simulink model "showKeyPoint"  (R2015a)
settings: Solver=ode45  StartTime=0.0  StopTime=10.0  RelTol=1e-3
InitFcn:
  | %% DSPBuilder Start
  | alt_dspbuilder_update_model(bdroot)
  | %% DSPBuilder End
libraries: allblocks_alteradspbuilder2 x340
(part 2 of 5)

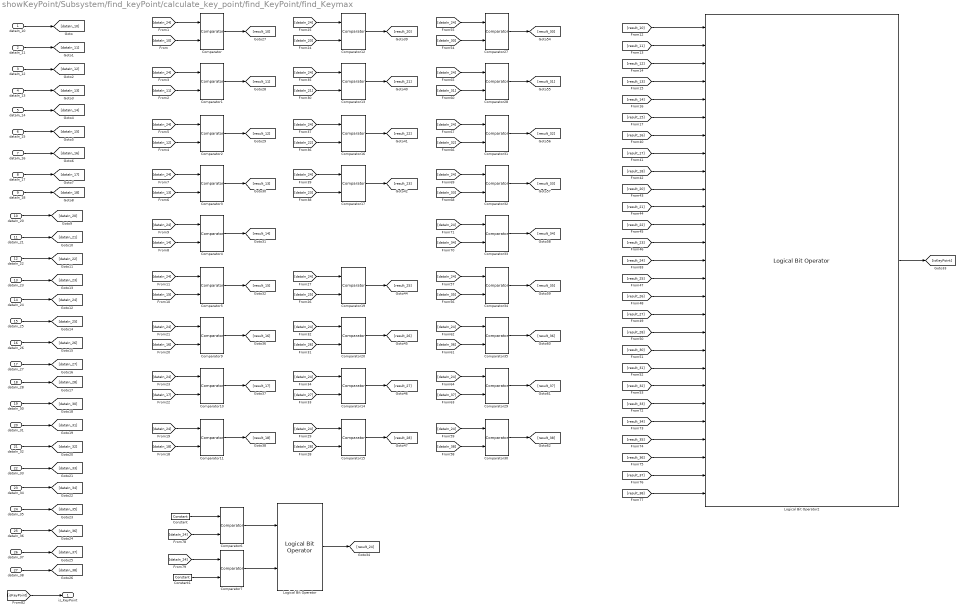
== system showKeyPoint/Subsystem/find_keyPoint/calculate_key_point/find_KeyPoint/find_Keymax ==
  dataIn_10 : Inport
  dataIn_11 : Inport  Port=2
  dataIn_12 : Inport  Port=3
  dataIn_13 : Inport  Port=4
  dataIn_14 : Inport  Port=5
  dataIn_15 : Inport  Port=6
  dataIn_16 : Inport  Port=7
  dataIn_17 : Inport  Port=8
  dataIn_18 : Inport  Port=9
  dataIn_20 : Inport  Port=10
  dataIn_21 : Inport  Port=11
  dataIn_22 : Inport  Port=12
  dataIn_23 : Inport  Port=13
  dataIn_24 : Inport  Port=14
  dataIn_25 : Inport  Port=15
  dataIn_26 : Inport  Port=16
  dataIn_27 : Inport  Port=17
  dataIn_28 : Inport  Port=18
  dataIn_30 : Inport  Port=19
  dataIn_31 : Inport  Port=20
  dataIn_32 : Inport  Port=21
  dataIn_33 : Inport  Port=22
  dataIn_34 : Inport  Port=23
  dataIn_35 : Inport  Port=24
  dataIn_36 : Inport  Port=25
  dataIn_37 : Inport  Port=26
  dataIn_38 : Inport  Port=27
  Comparator : allblocks_alteradspbuilder2/Comparator  direction=a > b  pipeline_display=0  allowFloatingPointOverride=on  logOutputs=off  logFile=C:\Users\ASUS\Desktop\sift_fpga_final\Gaussian filter 5x5\tb_gauss\gauss_Subsystem_find%5FkeyPoint_calculate%5Fkey%5Fpoint_find%5FKeyPoint_find%5FKeymax_Comparator.fixedpointlog
  Comparator1 : allblocks_alteradspbuilder2/Comparator  direction=a > b  pipeline_display=0  allowFloatingPointOverride=on  logOutputs=off  logFile=C:\Users\ASUS\Desktop\sift_fpga_final\Gaussian filter 5x5\tb_gauss\gauss_Subsystem_find%5FkeyPoint_calculate%5Fkey%5Fpoint_find%5FKeyPoint_find%5FKeymax_Comparator1.fixedpointlog
  Comparator10 : allblocks_alteradspbuilder2/Comparator  direction=a > b  pipeline_display=0  allowFloatingPointOverride=on  logOutputs=off  logFile=C:\Users\ASUS\Desktop\sift_fpga_final\Gaussian filter 5x5\tb_gauss\gauss_Subsystem_find%5FkeyPoint_calculate%5Fkey%5Fpoint_find%5FKeyPoint_find%5FKeymax_Comparator10.fixedpointlog
  Comparator11 : allblocks_alteradspbuilder2/Comparator  direction=a > b  pipeline_display=0  allowFloatingPointOverride=on  logOutputs=off  logFile=C:\Users\ASUS\Desktop\sift_fpga_final\Gaussian filter 5x5\tb_gauss\gauss_Subsystem_find%5FkeyPoint_calculate%5Fkey%5Fpoint_find%5FKeyPoint_find%5FKeymax_Comparator11.fixedpointlog
  Comparator12 : allblocks_alteradspbuilder2/Comparator  direction=a > b  pipeline_display=0  allowFloatingPointOverride=on  logOutputs=off  logFile=C:\Users\ASUS\Desktop\sift_fpga_final\Gaussian filter 5x5\tb_gauss\gauss_Subsystem_find%5FkeyPoint_calculate%5Fkey%5Fpoint_find%5FKeyPoint_find%5FKeymax_Comparator12.fixedpointlog
  Comparator13 : allblocks_alteradspbuilder2/Comparator  direction=a > b  pipeline_display=0  allowFloatingPointOverride=on  logOutputs=off  logFile=C:\Users\ASUS\Desktop\sift_fpga_final\Gaussian filter 5x5\tb_gauss\gauss_Subsystem_find%5FkeyPoint_calculate%5Fkey%5Fpoint_find%5FKeyPoint_find%5FKeymax_Comparator13.fixedpointlog
  Comparator14 : allblocks_alteradspbuilder2/Comparator  direction=a > b  pipeline_display=0  allowFloatingPointOverride=on  logOutputs=off  logFile=C:\Users\ASUS\Desktop\sift_fpga_final\Gaussian filter 5x5\tb_gauss\gauss_Subsystem_find%5FkeyPoint_calculate%5Fkey%5Fpoint_find%5FKeyPoint_find%5FKeymax_Comparator14.fixedpointlog
  Comparator15 : allblocks_alteradspbuilder2/Comparator  direction=a > b  pipeline_display=0  allowFloatingPointOverride=on  logOutputs=off  logFile=C:\Users\ASUS\Desktop\sift_fpga_final\Gaussian filter 5x5\tb_gauss\gauss_Subsystem_find%5FkeyPoint_calculate%5Fkey%5Fpoint_find%5FKeyPoint_find%5FKeymax_Comparator15.fixedpointlog
  Comparator16 : allblocks_alteradspbuilder2/Comparator  direction=a > b  pipeline_display=0  allowFloatingPointOverride=on  logOutputs=off  logFile=C:\Users\ASUS\Desktop\sift_fpga_final\Gaussian filter 5x5\tb_gauss\gauss_Subsystem_find%5FkeyPoint_calculate%5Fkey%5Fpoint_find%5FKeyPoint_find%5FKeymax_Comparator16.fixedpointlog
  Comparator17 : allblocks_alteradspbuilder2/Comparator  direction=a > b  pipeline_display=0  allowFloatingPointOverride=on  logOutputs=off  logFile=C:\Users\ASUS\Desktop\sift_fpga_final\Gaussian filter 5x5\tb_gauss\gauss_Subsystem_find%5FkeyPoint_calculate%5Fkey%5Fpoint_find%5FKeyPoint_find%5FKeymax_Comparator17.fixedpointlog
  Comparator19 : allblocks_alteradspbuilder2/Comparator  direction=a > b  pipeline_display=0  allowFloatingPointOverride=on  logOutputs=off  logFile=C:\Users\ASUS\Desktop\sift_fpga_final\Gaussian filter 5x5\tb_gauss\gauss_Subsystem_find%5FkeyPoint_calculate%5Fkey%5Fpoint_find%5FKeyPoint_find%5FKeymax_Comparator19.fixedpointlog
  Comparator2 : allblocks_alteradspbuilder2/Comparator  direction=a > b  pipeline_display=0  allowFloatingPointOverride=on  logOutputs=off  logFile=C:\Users\ASUS\Desktop\sift_fpga_final\Gaussian filter 5x5\tb_gauss\gauss_Subsystem_find%5FkeyPoint_calculate%5Fkey%5Fpoint_find%5FKeyPoint_find%5FKeymax_Comparator2.fixedpointlog
  Comparator20 : allblocks_alteradspbuilder2/Comparator  direction=a > b  pipeline_display=0  allowFloatingPointOverride=on  logOutputs=off  logFile=C:\Users\ASUS\Desktop\sift_fpga_final\Gaussian filter 5x5\tb_gauss\gauss_Subsystem_find%5FkeyPoint_calculate%5Fkey%5Fpoint_find%5FKeyPoint_find%5FKeymax_Comparator20.fixedpointlog
  Comparator27 : allblocks_alteradspbuilder2/Comparator  direction=a > b  pipeline_display=0  allowFloatingPointOverride=on  logOutputs=off  logFile=C:\Users\ASUS\Desktop\sift_fpga_final\Gaussian filter 5x5\tb_gauss\gauss_Subsystem_find%5FkeyPoint_calculate%5Fkey%5Fpoint_find%5FKeyPoint_find%5FKeymax_Comparator27.fixedpointlog
  Comparator28 : allblocks_alteradspbuilder2/Comparator  direction=a > b  pipeline_display=0  allowFloatingPointOverride=on  logOutputs=off  logFile=C:\Users\ASUS\Desktop\sift_fpga_final\Gaussian filter 5x5\tb_gauss\gauss_Subsystem_find%5FkeyPoint_calculate%5Fkey%5Fpoint_find%5FKeyPoint_find%5FKeymax_Comparator28.fixedpointlog
  Comparator29 : allblocks_alteradspbuilder2/Comparator  direction=a > b  pipeline_display=0  allowFloatingPointOverride=on  logOutputs=off  logFile=C:\Users\ASUS\Desktop\sift_fpga_final\Gaussian filter 5x5\tb_gauss\gauss_Subsystem_find%5FkeyPoint_calculate%5Fkey%5Fpoint_find%5FKeyPoint_find%5FKeymax_Comparator29.fixedpointlog
  Comparator3 : allblocks_alteradspbuilder2/Comparator  direction=a > b  pipeline_display=0  allowFloatingPointOverride=on  logOutputs=off  logFile=C:\Users\ASUS\Desktop\sift_fpga_final\Gaussian filter 5x5\tb_gauss\gauss_Subsystem_find%5FkeyPoint_calculate%5Fkey%5Fpoint_find%5FKeyPoint_find%5FKeymax_Comparator3.fixedpointlog
  Comparator30 : allblocks_alteradspbuilder2/Comparator  direction=a > b  pipeline_display=0  allowFloatingPointOverride=on  logOutputs=off  logFile=C:\Users\ASUS\Desktop\sift_fpga_final\Gaussian filter 5x5\tb_gauss\gauss_Subsystem_find%5FkeyPoint_calculate%5Fkey%5Fpoint_find%5FKeyPoint_find%5FKeymax_Comparator30.fixedpointlog
  Comparator31 : allblocks_alteradspbuilder2/Comparator  direction=a > b  pipeline_display=0  allowFloatingPointOverride=on  logOutputs=off  logFile=C:\Users\ASUS\Desktop\sift_fpga_final\Gaussian filter 5x5\tb_gauss\gauss_Subsystem_find%5FkeyPoint_calculate%5Fkey%5Fpoint_find%5FKeyPoint_find%5FKeymax_Comparator31.fixedpointlog
  Comparator32 : allblocks_alteradspbuilder2/Comparator  direction=a > b  pipeline_display=0  allowFloatingPointOverride=on  logOutputs=off  logFile=C:\Users\ASUS\Desktop\sift_fpga_final\Gaussian filter 5x5\tb_gauss\gauss_Subsystem_find%5FkeyPoint_calculate%5Fkey%5Fpoint_find%5FKeyPoint_find%5FKeymax_Comparator32.fixedpointlog
  Comparator33 : allblocks_alteradspbuilder2/Comparator  direction=a > b  pipeline_display=0  allowFloatingPointOverride=on  logOutputs=off  logFile=C:\Users\ASUS\Desktop\sift_fpga_final\Gaussian filter 5x5\tb_gauss\gauss_Subsystem_find%5FkeyPoint_calculate%5Fkey%5Fpoint_find%5FKeyPoint_find%5FKeymax_Comparator33.fixedpointlog
  Comparator34 : allblocks_alteradspbuilder2/Comparator  direction=a > b  pipeline_display=0  allowFloatingPointOverride=on  logOutputs=off  logFile=C:\Users\ASUS\Desktop\sift_fpga_final\Gaussian filter 5x5\tb_gauss\gauss_Subsystem_find%5FkeyPoint_calculate%5Fkey%5Fpoint_find%5FKeyPoint_find%5FKeymax_Comparator34.fixedpointlog
  Comparator35 : allblocks_alteradspbuilder2/Comparator  direction=a > b  pipeline_display=0  allowFloatingPointOverride=on  logOutputs=off  logFile=C:\Users\ASUS\Desktop\sift_fpga_final\Gaussian filter 5x5\tb_gauss\gauss_Subsystem_find%5FkeyPoint_calculate%5Fkey%5Fpoint_find%5FKeyPoint_find%5FKeymax_Comparator35.fixedpointlog
  Comparator4 : allblocks_alteradspbuilder2/Comparator  direction=a > b  pipeline_display=0  allowFloatingPointOverride=on  logOutputs=off  logFile=C:\Users\ASUS\Desktop\sift_fpga_final\Gaussian filter 5x5\tb_gauss\gauss_Subsystem_find%5FkeyPoint_calculate%5Fkey%5Fpoint_find%5FKeyPoint_find%5FKeymax_Comparator4.fixedpointlog
  Comparator5 : allblocks_alteradspbuilder2/Comparator  direction=a > b  pipeline_display=0  allowFloatingPointOverride=on  logOutputs=off  logFile=C:\Users\ASUS\Desktop\sift_fpga_final\Gaussian filter 5x5\tb_gauss\gauss_Subsystem_find%5FkeyPoint_calculate%5Fkey%5Fpoint_find%5FKeyPoint_find%5FKeymax_Comparator5.fixedpointlog
  Comparator6 : allblocks_alteradspbuilder2/Comparator  direction=a < b  pipeline_display=0  allowFloatingPointOverride=on  logOutputs=off  logFile=C:\Users\ASUS\Desktop\sift_fpga_final\Gaussian filter 5x5\tb_gauss\gauss_Subsystem_find%5FkeyPoint_calculate%5Fkey%5Fpoint_find%5FKeyPoint_find%5FKeymax_Comparator6.fixedpointlog
  Comparator7 : allblocks_alteradspbuilder2/Comparator  direction=a < b  pipeline_display=0  allowFloatingPointOverride=on  logOutputs=off  logFile=C:\Users\ASUS\Desktop\sift_fpga_final\Gaussian filter 5x5\tb_gauss\gauss_Subsystem_find%5FkeyPoint_calculate%5Fkey%5Fpoint_find%5FKeyPoint_find%5FKeymax_Comparator7.fixedpointlog
  Comparator9 : allblocks_alteradspbuilder2/Comparator  direction=a > b  pipeline_display=0  allowFloatingPointOverride=on  logOutputs=off  logFile=C:\Users\ASUS\Desktop\sift_fpga_final\Gaussian filter 5x5\tb_gauss\gauss_Subsystem_find%5FkeyPoint_calculate%5Fkey%5Fpoint_find%5FKeyPoint_find%5FKeymax_Comparator9.fixedpointlog
  Constant : allblocks_alteradspbuilder2/Constant  mask_cst=0.8*0.015  BusType=Signed Fractional  bwl=9  bwr=16  roundMode=Truncate  satMode=Wrap  SpecifyClock=off  allowFloatingPointOverride=on  logOutputs=off  logFile=C:\Users\ASUS\Desktop\sift_fpga_final\Gaussian filter 5x5\tb_gauss\gauss_Subsystem_find%5FkeyPoint_calculate%5Fkey%5Fpoint_find%5FKeyPoint_find%5FKeymax_Constant.fixedpointlog
  Constant1 : allblocks_alteradspbuilder2/Constant  mask_cst=-0.8*0.015  BusType=Signed Fractional  bwl=9  bwr=16  roundMode=Truncate  satMode=Wrap  SpecifyClock=off  allowFloatingPointOverride=on  logOutputs=off  logFile=C:\Users\ASUS\Desktop\sift_fpga_final\Gaussian filter 5x5\tb_gauss\gauss_Subsystem_find%5FkeyPoint_calculate%5Fkey%5Fpoint_find%5FKeyPoint_find%5FKeymax_Constant1.fixedpointlog
  Logical Bit Operator : allblocks_alteradspbuilder2/Logical Bit Operator  LogicalOperator=OR  user_inputs=2  pipeline_display=0
  Logical Bit Operator2 : allblocks_alteradspbuilder2/Logical Bit Operator  LogicalOperator=AND  user_inputs=27  pipeline_display=0
  is_KeyPoint : Outport
  wires:
  dataIn_18/1 -> [dataIn_18]
  dataIn_10/1 -> [dataIn_10]
  [result_10] -> Logical Bit Operator2/1
  [dataIn_24] -> Comparator/1
  Comparator1/1 -> [result_11]
  [dataIn_10] -> Comparator/2
  [dataIn_24] -> Comparator1/1
  [dataIn_11] -> Comparator1/2
  [result_20] -> Logical Bit Operator2/10
  [result_11] -> Logical Bit Operator2/2
  [result_22] -> Logical Bit Operator2/12
  [result_23] -> Logical Bit Operator2/13
  Comparator7/1 -> Logical Bit Operator/2
  [dataIn_24] -> Comparator2/1
  [dataIn_24] -> Comparator6/2
  Comparator2/1 -> [result_12]
  [dataIn_12] -> Comparator2/2
  [result_21] -> Logical Bit Operator2/11
  [dataIn_24] -> Comparator9/1
  Comparator9/1 -> [result_16]
  [dataIn_24] -> Comparator10/1
  [dataIn_16] -> Comparator9/2
  Comparator10/1 -> [result_17]
  [dataIn_17] -> Comparator10/2
  [dataIn_24] -> Comparator11/1
  Comparator11/1 -> [result_18]
  [dataIn_18] -> Comparator11/2
  dataIn_14/1 -> [dataIn_14]
  dataIn_15/1 -> [dataIn_15]
  dataIn_17/1 -> [dataIn_17]
  dataIn_16/1 -> [dataIn_16]
  dataIn_24/1 -> [dataIn_24]
  dataIn_27/1 -> [dataIn_27]
  dataIn_28/1 -> [dataIn_28]
  dataIn_25/1 -> [dataIn_25]
  dataIn_22/1 -> [dataIn_22]
  dataIn_20/1 -> [dataIn_20]
  dataIn_21/1 -> [dataIn_21]
  dataIn_23/1 -> [dataIn_23]
  dataIn_26/1 -> [dataIn_26]
  dataIn_30/1 -> [dataIn_30]
  dataIn_31/1 -> [dataIn_31]
  dataIn_32/1 -> [dataIn_32]
  dataIn_33/1 -> [dataIn_33]
  dataIn_37/1 -> [dataIn_37]
  dataIn_35/1 -> [dataIn_35]
  dataIn_34/1 -> [dataIn_34]
  dataIn_36/1 -> [dataIn_36]
  dataIn_38/1 -> [dataIn_38]
  dataIn_11/1 -> [dataIn_11]
  [dataIn_24] -> Comparator7/1
  [dataIn_13] -> Comparator3/2
  Comparator3/1 -> [result_13]
  [dataIn_24] -> Comparator4/1
  [dataIn_24] -> Comparator3/1
  [dataIn_24] -> Comparator5/1
  Comparator5/1 -> [result_15]
  [dataIn_14] -> Comparator4/2
  [dataIn_15] -> Comparator5/2
  Comparator4/1 -> [result_14]
  [dataIn_24] -> Comparator27/1
  [dataIn_24] -> Comparator28/1
  [dataIn_24] -> Comparator31/1
  [dataIn_32] -> Comparator31/2
  [dataIn_24] -> Comparator32/1
  [dataIn_33] -> Comparator32/2
  [dataIn_24] -> Comparator33/1
  Comparator32/1 -> [result_33]
  Comparator27/1 -> [result_30]
  Comparator28/1 -> [result_31]
  Comparator31/1 -> [result_32]
  [dataIn_30] -> Comparator27/2
  [dataIn_31] -> Comparator28/2
  [dataIn_35] -> Comparator34/2
  Comparator35/1 -> [result_36]
  Comparator34/1 -> [result_35]
  [dataIn_34] -> Comparator33/2
  [dataIn_24] -> Comparator35/1
  Comparator29/1 -> [result_37]
  [dataIn_24] -> Comparator30/1
  [dataIn_36] -> Comparator35/2
  Comparator30/1 -> [result_38]
  [dataIn_24] -> Comparator34/1
  [dataIn_24] -> Comparator29/1
  [dataIn_37] -> Comparator29/2
  [dataIn_38] -> Comparator30/2
  Comparator33/1 -> [result_34]
  [result_13] -> Logical Bit Operator2/4
  [result_17] -> Logical Bit Operator2/8
  [result_14] -> Logical Bit Operator2/5
  [result_15] -> Logical Bit Operator2/6
  [result_16] -> Logical Bit Operator2/7
  [result_18] -> Logical Bit Operator2/9
  [result_12] -> Logical Bit Operator2/3
  Constant/1 -> Comparator6/1
  Logical Bit Operator/1 -> [result_24]
  Logical Bit Operator2/1 -> [isKeyPoint]
  Constant1/1 -> Comparator7/2
  Comparator6/1 -> Logical Bit Operator/1
  [dataIn_24] -> Comparator12/1
  [dataIn_25] -> Comparator19/2
  Comparator13/1 -> [result_21]
  Comparator19/1 -> [result_25]
  [dataIn_24] -> Comparator19/1
  [dataIn_20] -> Comparator12/2
  [dataIn_24] -> Comparator16/1
  [dataIn_24] -> Comparator14/1
  [dataIn_24] -> Comparator13/1
  Comparator16/1 -> [result_22]
  [dataIn_22] -> Comparator16/2
  Comparator14/1 -> [result_27]
  [dataIn_24] -> Comparator17/1
  [dataIn_23] -> Comparator17/2
  [dataIn_24] -> Comparator15/1
  [dataIn_27] -> Comparator14/2
  Comparator17/1 -> [result_23]
  [dataIn_28] -> Comparator15/2
  [dataIn_26] -> Comparator20/2
  Comparator12/1 -> [result_20]
  [dataIn_24] -> Comparator20/1
  Comparator15/1 -> [result_28]
  Comparator20/1 -> [result_26]
  [dataIn_21] -> Comparator13/2
  [isKeyPoint] -> is_KeyPoint/1
  dataIn_12/1 -> [dataIn_12]
  dataIn_13/1 -> [dataIn_13]
  Comparator/1 -> [result_10]
  [result_28] -> Logical Bit Operator2/18
  [result_30] -> Logical Bit Operator2/19
  [result_31] -> Logical Bit Operator2/20
  [result_33] -> Logical Bit Operator2/22
  [result_34] -> Logical Bit Operator2/23
  [result_36] -> Logical Bit Operator2/25
  [result_35] -> Logical Bit Operator2/24
  [result_32] -> Logical Bit Operator2/21
  [result_37] -> Logical Bit Operator2/26
  [result_38] -> Logical Bit Operator2/27
  [result_26] -> Logical Bit Operator2/16
  [result_25] -> Logical Bit Operator2/15
  [result_27] -> Logical Bit Operator2/17
  [result_24] -> Logical Bit Operator2/14

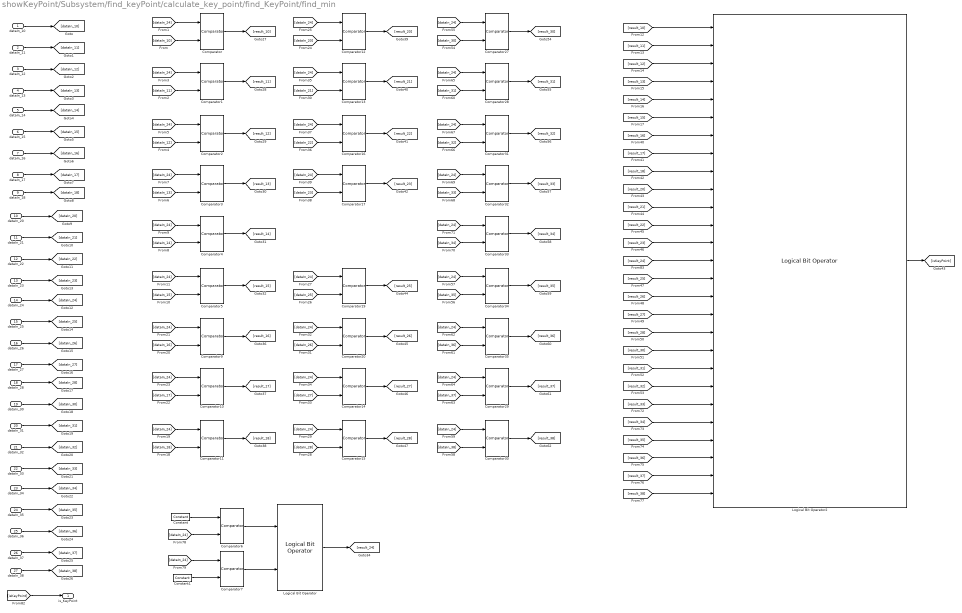
== system showKeyPoint/Subsystem/find_keyPoint/calculate_key_point/find_KeyPoint/find_min ==
  dataIn_10 : Inport
  dataIn_11 : Inport  Port=2
  dataIn_12 : Inport  Port=3
  dataIn_13 : Inport  Port=4
  dataIn_14 : Inport  Port=5
  dataIn_15 : Inport  Port=6
  dataIn_16 : Inport  Port=7
  dataIn_17 : Inport  Port=8
  dataIn_18 : Inport  Port=9
  dataIn_20 : Inport  Port=10
  dataIn_21 : Inport  Port=11
  dataIn_22 : Inport  Port=12
  dataIn_23 : Inport  Port=13
  dataIn_24 : Inport  Port=14
  dataIn_25 : Inport  Port=15
  dataIn_26 : Inport  Port=16
  dataIn_27 : Inport  Port=17
  dataIn_28 : Inport  Port=18
  dataIn_30 : Inport  Port=19
  dataIn_31 : Inport  Port=20
  dataIn_32 : Inport  Port=21
  dataIn_33 : Inport  Port=22
  dataIn_34 : Inport  Port=23
  dataIn_35 : Inport  Port=24
  dataIn_36 : Inport  Port=25
  dataIn_37 : Inport  Port=26
  dataIn_38 : Inport  Port=27
  Comparator : allblocks_alteradspbuilder2/Comparator  direction=a < b  pipeline_display=0  allowFloatingPointOverride=on  logOutputs=off  logFile=C:\Users\ASUS\Desktop\sift_fpga_final\Gaussian filter 5x5\tb_gauss\gauss_Subsystem_find%5FkeyPoint_calculate%5Fkey%5Fpoint_find%5FKeyPoint_find%5Fmin_Comparator.fixedpointlog
  Comparator1 : allblocks_alteradspbuilder2/Comparator  direction=a < b  pipeline_display=0  allowFloatingPointOverride=on  logOutputs=off  logFile=C:\Users\ASUS\Desktop\sift_fpga_final\Gaussian filter 5x5\tb_gauss\gauss_Subsystem_find%5FkeyPoint_calculate%5Fkey%5Fpoint_find%5FKeyPoint_find%5Fmin_Comparator1.fixedpointlog
  Comparator10 : allblocks_alteradspbuilder2/Comparator  direction=a < b  pipeline_display=0  allowFloatingPointOverride=on  logOutputs=off  logFile=C:\Users\ASUS\Desktop\sift_fpga_final\Gaussian filter 5x5\tb_gauss\gauss_Subsystem_find%5FkeyPoint_calculate%5Fkey%5Fpoint_find%5FKeyPoint_find%5Fmin_Comparator10.fixedpointlog
  Comparator11 : allblocks_alteradspbuilder2/Comparator  direction=a < b  pipeline_display=0  allowFloatingPointOverride=on  logOutputs=off  logFile=C:\Users\ASUS\Desktop\sift_fpga_final\Gaussian filter 5x5\tb_gauss\gauss_Subsystem_find%5FkeyPoint_calculate%5Fkey%5Fpoint_find%5FKeyPoint_find%5Fmin_Comparator11.fixedpointlog
  Comparator12 : allblocks_alteradspbuilder2/Comparator  direction=a < b  pipeline_display=0  allowFloatingPointOverride=on  logOutputs=off  logFile=C:\Users\ASUS\Desktop\sift_fpga_final\Gaussian filter 5x5\tb_gauss\gauss_Subsystem_find%5FkeyPoint_calculate%5Fkey%5Fpoint_find%5FKeyPoint_find%5Fmin_Comparator12.fixedpointlog
  Comparator13 : allblocks_alteradspbuilder2/Comparator  direction=a < b  pipeline_display=0  allowFloatingPointOverride=on  logOutputs=off  logFile=C:\Users\ASUS\Desktop\sift_fpga_final\Gaussian filter 5x5\tb_gauss\gauss_Subsystem_find%5FkeyPoint_calculate%5Fkey%5Fpoint_find%5FKeyPoint_find%5Fmin_Comparator13.fixedpointlog
  Comparator14 : allblocks_alteradspbuilder2/Comparator  direction=a < b  pipeline_display=0  allowFloatingPointOverride=on  logOutputs=off  logFile=C:\Users\ASUS\Desktop\sift_fpga_final\Gaussian filter 5x5\tb_gauss\gauss_Subsystem_find%5FkeyPoint_calculate%5Fkey%5Fpoint_find%5FKeyPoint_find%5Fmin_Comparator14.fixedpointlog
  Comparator15 : allblocks_alteradspbuilder2/Comparator  direction=a < b  pipeline_display=0  allowFloatingPointOverride=on  logOutputs=off  logFile=C:\Users\ASUS\Desktop\sift_fpga_final\Gaussian filter 5x5\tb_gauss\gauss_Subsystem_find%5FkeyPoint_calculate%5Fkey%5Fpoint_find%5FKeyPoint_find%5Fmin_Comparator15.fixedpointlog
  Comparator16 : allblocks_alteradspbuilder2/Comparator  direction=a < b  pipeline_display=0  allowFloatingPointOverride=on  logOutputs=off  logFile=C:\Users\ASUS\Desktop\sift_fpga_final\Gaussian filter 5x5\tb_gauss\gauss_Subsystem_find%5FkeyPoint_calculate%5Fkey%5Fpoint_find%5FKeyPoint_find%5Fmin_Comparator16.fixedpointlog
  Comparator17 : allblocks_alteradspbuilder2/Comparator  direction=a < b  pipeline_display=0  allowFloatingPointOverride=on  logOutputs=off  logFile=C:\Users\ASUS\Desktop\sift_fpga_final\Gaussian filter 5x5\tb_gauss\gauss_Subsystem_find%5FkeyPoint_calculate%5Fkey%5Fpoint_find%5FKeyPoint_find%5Fmin_Comparator17.fixedpointlog
  Comparator19 : allblocks_alteradspbuilder2/Comparator  direction=a < b  pipeline_display=0  allowFloatingPointOverride=on  logOutputs=off  logFile=C:\Users\ASUS\Desktop\sift_fpga_final\Gaussian filter 5x5\tb_gauss\gauss_Subsystem_find%5FkeyPoint_calculate%5Fkey%5Fpoint_find%5FKeyPoint_find%5Fmin_Comparator19.fixedpointlog
  Comparator2 : allblocks_alteradspbuilder2/Comparator  direction=a < b  pipeline_display=0  allowFloatingPointOverride=on  logOutputs=off  logFile=C:\Users\ASUS\Desktop\sift_fpga_final\Gaussian filter 5x5\tb_gauss\gauss_Subsystem_find%5FkeyPoint_calculate%5Fkey%5Fpoint_find%5FKeyPoint_find%5Fmin_Comparator2.fixedpointlog
  Comparator20 : allblocks_alteradspbuilder2/Comparator  direction=a < b  pipeline_display=0  allowFloatingPointOverride=on  logOutputs=off  logFile=C:\Users\ASUS\Desktop\sift_fpga_final\Gaussian filter 5x5\tb_gauss\gauss_Subsystem_find%5FkeyPoint_calculate%5Fkey%5Fpoint_find%5FKeyPoint_find%5Fmin_Comparator20.fixedpointlog
  Comparator27 : allblocks_alteradspbuilder2/Comparator  direction=a < b  pipeline_display=0  allowFloatingPointOverride=on  logOutputs=off  logFile=C:\Users\ASUS\Desktop\sift_fpga_final\Gaussian filter 5x5\tb_gauss\gauss_Subsystem_find%5FkeyPoint_calculate%5Fkey%5Fpoint_find%5FKeyPoint_find%5Fmin_Comparator27.fixedpointlog
  Comparator28 : allblocks_alteradspbuilder2/Comparator  direction=a < b  pipeline_display=0  allowFloatingPointOverride=on  logOutputs=off  logFile=C:\Users\ASUS\Desktop\sift_fpga_final\Gaussian filter 5x5\tb_gauss\gauss_Subsystem_find%5FkeyPoint_calculate%5Fkey%5Fpoint_find%5FKeyPoint_find%5Fmin_Comparator28.fixedpointlog
  Comparator29 : allblocks_alteradspbuilder2/Comparator  direction=a < b  pipeline_display=0  allowFloatingPointOverride=on  logOutputs=off  logFile=C:\Users\ASUS\Desktop\sift_fpga_final\Gaussian filter 5x5\tb_gauss\gauss_Subsystem_find%5FkeyPoint_calculate%5Fkey%5Fpoint_find%5FKeyPoint_find%5Fmin_Comparator29.fixedpointlog
  Comparator3 : allblocks_alteradspbuilder2/Comparator  direction=a < b  pipeline_display=0  allowFloatingPointOverride=on  logOutputs=off  logFile=C:\Users\ASUS\Desktop\sift_fpga_final\Gaussian filter 5x5\tb_gauss\gauss_Subsystem_find%5FkeyPoint_calculate%5Fkey%5Fpoint_find%5FKeyPoint_find%5Fmin_Comparator3.fixedpointlog
  Comparator30 : allblocks_alteradspbuilder2/Comparator  direction=a < b  pipeline_display=0  allowFloatingPointOverride=on  logOutputs=off  logFile=C:\Users\ASUS\Desktop\sift_fpga_final\Gaussian filter 5x5\tb_gauss\gauss_Subsystem_find%5FkeyPoint_calculate%5Fkey%5Fpoint_find%5FKeyPoint_find%5Fmin_Comparator30.fixedpointlog
  Comparator31 : allblocks_alteradspbuilder2/Comparator  direction=a < b  pipeline_display=0  allowFloatingPointOverride=on  logOutputs=off  logFile=C:\Users\ASUS\Desktop\sift_fpga_final\Gaussian filter 5x5\tb_gauss\gauss_Subsystem_find%5FkeyPoint_calculate%5Fkey%5Fpoint_find%5FKeyPoint_find%5Fmin_Comparator31.fixedpointlog
  Comparator32 : allblocks_alteradspbuilder2/Comparator  direction=a < b  pipeline_display=0  allowFloatingPointOverride=on  logOutputs=off  logFile=C:\Users\ASUS\Desktop\sift_fpga_final\Gaussian filter 5x5\tb_gauss\gauss_Subsystem_find%5FkeyPoint_calculate%5Fkey%5Fpoint_find%5FKeyPoint_find%5Fmin_Comparator32.fixedpointlog
  Comparator33 : allblocks_alteradspbuilder2/Comparator  direction=a < b  pipeline_display=0  allowFloatingPointOverride=on  logOutputs=off  logFile=C:\Users\ASUS\Desktop\sift_fpga_final\Gaussian filter 5x5\tb_gauss\gauss_Subsystem_find%5FkeyPoint_calculate%5Fkey%5Fpoint_find%5FKeyPoint_find%5Fmin_Comparator33.fixedpointlog
  Comparator34 : allblocks_alteradspbuilder2/Comparator  direction=a < b  pipeline_display=0  allowFloatingPointOverride=on  logOutputs=off  logFile=C:\Users\ASUS\Desktop\sift_fpga_final\Gaussian filter 5x5\tb_gauss\gauss_Subsystem_find%5FkeyPoint_calculate%5Fkey%5Fpoint_find%5FKeyPoint_find%5Fmin_Comparator34.fixedpointlog
  Comparator35 : allblocks_alteradspbuilder2/Comparator  direction=a < b  pipeline_display=0  allowFloatingPointOverride=on  logOutputs=off  logFile=C:\Users\ASUS\Desktop\sift_fpga_final\Gaussian filter 5x5\tb_gauss\gauss_Subsystem_find%5FkeyPoint_calculate%5Fkey%5Fpoint_find%5FKeyPoint_find%5Fmin_Comparator35.fixedpointlog
  Comparator4 : allblocks_alteradspbuilder2/Comparator  direction=a < b  pipeline_display=0  allowFloatingPointOverride=on  logOutputs=off  logFile=C:\Users\ASUS\Desktop\sift_fpga_final\Gaussian filter 5x5\tb_gauss\gauss_Subsystem_find%5FkeyPoint_calculate%5Fkey%5Fpoint_find%5FKeyPoint_find%5Fmin_Comparator4.fixedpointlog
  Comparator5 : allblocks_alteradspbuilder2/Comparator  direction=a < b  pipeline_display=0  allowFloatingPointOverride=on  logOutputs=off  logFile=C:\Users\ASUS\Desktop\sift_fpga_final\Gaussian filter 5x5\tb_gauss\gauss_Subsystem_find%5FkeyPoint_calculate%5Fkey%5Fpoint_find%5FKeyPoint_find%5Fmin_Comparator5.fixedpointlog
  Comparator6 : allblocks_alteradspbuilder2/Comparator  direction=a < b  pipeline_display=0  allowFloatingPointOverride=on  logOutputs=off  logFile=C:\Users\ASUS\Desktop\sift_fpga_final\Gaussian filter 5x5\tb_gauss\gauss_Subsystem_find%5FkeyPoint_calculate%5Fkey%5Fpoint_find%5FKeyPoint_find%5Fmin_Comparator6.fixedpointlog
  Comparator7 : allblocks_alteradspbuilder2/Comparator  direction=a < b  pipeline_display=0  allowFloatingPointOverride=on  logOutputs=off  logFile=C:\Users\ASUS\Desktop\sift_fpga_final\Gaussian filter 5x5\tb_gauss\gauss_Subsystem_find%5FkeyPoint_calculate%5Fkey%5Fpoint_find%5FKeyPoint_find%5Fmin_Comparator7.fixedpointlog
  Comparator9 : allblocks_alteradspbuilder2/Comparator  direction=a < b  pipeline_display=0  allowFloatingPointOverride=on  logOutputs=off  logFile=C:\Users\ASUS\Desktop\sift_fpga_final\Gaussian filter 5x5\tb_gauss\gauss_Subsystem_find%5FkeyPoint_calculate%5Fkey%5Fpoint_find%5FKeyPoint_find%5Fmin_Comparator9.fixedpointlog
  Constant : allblocks_alteradspbuilder2/Constant  mask_cst=0.8*0.015  BusType=Signed Fractional  bwl=9  bwr=16  roundMode=Truncate  satMode=Wrap  SpecifyClock=off  allowFloatingPointOverride=on  logOutputs=off  logFile=C:\Users\ASUS\Desktop\sift_fpga_final\Gaussian filter 5x5\tb_gauss\gauss_Subsystem_find%5FkeyPoint_calculate%5Fkey%5Fpoint_find%5FKeyPoint_find%5Fmin_Constant.fixedpointlog
  Constant1 : allblocks_alteradspbuilder2/Constant  mask_cst=-0.8*0.015  BusType=Signed Fractional  bwl=9  bwr=16  roundMode=Truncate  satMode=Wrap  SpecifyClock=off  allowFloatingPointOverride=on  logOutputs=off  logFile=C:\Users\ASUS\Desktop\sift_fpga_final\Gaussian filter 5x5\tb_gauss\gauss_Subsystem_find%5FkeyPoint_calculate%5Fkey%5Fpoint_find%5FKeyPoint_find%5Fmin_Constant1.fixedpointlog
  Logical Bit Operator : allblocks_alteradspbuilder2/Logical Bit Operator  LogicalOperator=OR  user_inputs=2  pipeline_display=0
  Logical Bit Operator2 : allblocks_alteradspbuilder2/Logical Bit Operator  LogicalOperator=AND  user_inputs=27  pipeline_display=0
  is_KeyPoint : Outport
  wires:
  dataIn_18/1 -> [dataIn_18]
  dataIn_10/1 -> [dataIn_10]
  [result_10] -> Logical Bit Operator2/1
  [dataIn_24] -> Comparator/1
  Comparator1/1 -> [result_11]
  [dataIn_10] -> Comparator/2
  [dataIn_24] -> Comparator1/1
  [dataIn_11] -> Comparator1/2
  [result_20] -> Logical Bit Operator2/10
  [result_11] -> Logical Bit Operator2/2
  [result_22] -> Logical Bit Operator2/12
  [result_23] -> Logical Bit Operator2/13
  Comparator7/1 -> Logical Bit Operator/2
  [dataIn_24] -> Comparator2/1
  [dataIn_24] -> Comparator6/2
  Comparator2/1 -> [result_12]
  [dataIn_12] -> Comparator2/2
  [result_21] -> Logical Bit Operator2/11
  [dataIn_24] -> Comparator9/1
  Comparator9/1 -> [result_16]
  [dataIn_24] -> Comparator10/1
  [dataIn_16] -> Comparator9/2
  Comparator10/1 -> [result_17]
  [dataIn_17] -> Comparator10/2
  [dataIn_24] -> Comparator11/1
  Comparator11/1 -> [result_18]
  [dataIn_18] -> Comparator11/2
  dataIn_14/1 -> [dataIn_14]
  dataIn_15/1 -> [dataIn_15]
  dataIn_17/1 -> [dataIn_17]
  dataIn_16/1 -> [dataIn_16]
  dataIn_24/1 -> [dataIn_24]
  dataIn_27/1 -> [dataIn_27]
  dataIn_28/1 -> [dataIn_28]
  dataIn_25/1 -> [dataIn_25]
  dataIn_22/1 -> [dataIn_22]
  dataIn_20/1 -> [dataIn_20]
  dataIn_21/1 -> [dataIn_21]
  dataIn_23/1 -> [dataIn_23]
  dataIn_26/1 -> [dataIn_26]
  dataIn_30/1 -> [dataIn_30]
  dataIn_31/1 -> [dataIn_31]
  dataIn_32/1 -> [dataIn_32]
  dataIn_33/1 -> [dataIn_33]
  dataIn_37/1 -> [dataIn_37]
  dataIn_35/1 -> [dataIn_35]
  dataIn_34/1 -> [dataIn_34]
  dataIn_36/1 -> [dataIn_36]
  dataIn_38/1 -> [dataIn_38]
  dataIn_11/1 -> [dataIn_11]
  [dataIn_24] -> Comparator7/1
  [dataIn_13] -> Comparator3/2
  Comparator3/1 -> [result_13]
  [dataIn_24] -> Comparator4/1
  [dataIn_24] -> Comparator3/1
  [dataIn_24] -> Comparator5/1
  Comparator5/1 -> [result_15]
  [dataIn_14] -> Comparator4/2
  [dataIn_15] -> Comparator5/2
  Comparator4/1 -> [result_14]
  [dataIn_24] -> Comparator27/1
  [dataIn_24] -> Comparator28/1
  [dataIn_24] -> Comparator31/1
  [dataIn_32] -> Comparator31/2
  [dataIn_24] -> Comparator32/1
  [dataIn_33] -> Comparator32/2
  [dataIn_24] -> Comparator33/1
  Comparator32/1 -> [result_33]
  Comparator27/1 -> [result_30]
  Comparator28/1 -> [result_31]
  Comparator31/1 -> [result_32]
  [dataIn_30] -> Comparator27/2
  [dataIn_31] -> Comparator28/2
  [dataIn_35] -> Comparator34/2
  Comparator35/1 -> [result_36]
  Comparator34/1 -> [result_35]
  [dataIn_34] -> Comparator33/2
  [dataIn_24] -> Comparator35/1
  Comparator29/1 -> [result_37]
  [dataIn_24] -> Comparator30/1
  [dataIn_36] -> Comparator35/2
  Comparator30/1 -> [result_38]
  [dataIn_24] -> Comparator34/1
  [dataIn_24] -> Comparator29/1
  [dataIn_37] -> Comparator29/2
  [dataIn_38] -> Comparator30/2
  Comparator33/1 -> [result_34]
  [result_13] -> Logical Bit Operator2/4
  [result_17] -> Logical Bit Operator2/8
  [result_14] -> Logical Bit Operator2/5
  [result_15] -> Logical Bit Operator2/6
  [result_16] -> Logical Bit Operator2/7
  [result_18] -> Logical Bit Operator2/9
  [result_12] -> Logical Bit Operator2/3
  Constant/1 -> Comparator6/1
  Logical Bit Operator/1 -> [result_24]
  Constant1/1 -> Comparator7/2
  Comparator6/1 -> Logical Bit Operator/1
  [dataIn_24] -> Comparator12/1
  [dataIn_25] -> Comparator19/2
  Comparator13/1 -> [result_21]
  Comparator19/1 -> [result_25]
  [dataIn_24] -> Comparator19/1
  [dataIn_20] -> Comparator12/2
  [dataIn_24] -> Comparator16/1
  [dataIn_24] -> Comparator14/1
  [dataIn_24] -> Comparator13/1
  Comparator16/1 -> [result_22]
  [dataIn_22] -> Comparator16/2
  Comparator14/1 -> [result_27]
  [dataIn_24] -> Comparator17/1
  [dataIn_23] -> Comparator17/2
  [dataIn_24] -> Comparator15/1
  [dataIn_27] -> Comparator14/2
  Comparator17/1 -> [result_23]
  [dataIn_28] -> Comparator15/2
  [dataIn_26] -> Comparator20/2
  Comparator12/1 -> [result_20]
  [dataIn_24] -> Comparator20/1
  Comparator15/1 -> [result_28]
  Comparator20/1 -> [result_26]
  [dataIn_21] -> Comparator13/2
  [isKeyPoint] -> is_KeyPoint/1
  dataIn_12/1 -> [dataIn_12]
  dataIn_13/1 -> [dataIn_13]
  Comparator/1 -> [result_10]
  [result_28] -> Logical Bit Operator2/18
  [result_30] -> Logical Bit Operator2/19
  [result_31] -> Logical Bit Operator2/20
  [result_33] -> Logical Bit Operator2/22
  [result_34] -> Logical Bit Operator2/23
  [result_36] -> Logical Bit Operator2/25
  [result_35] -> Logical Bit Operator2/24
  [result_32] -> Logical Bit Operator2/21
  [result_37] -> Logical Bit Operator2/26
  [result_38] -> Logical Bit Operator2/27
  [result_26] -> Logical Bit Operator2/16
  [result_25] -> Logical Bit Operator2/15
  [result_27] -> Logical Bit Operator2/17
  [result_24] -> Logical Bit Operator2/14
  Logical Bit Operator2/1 -> [isKeyPoint]

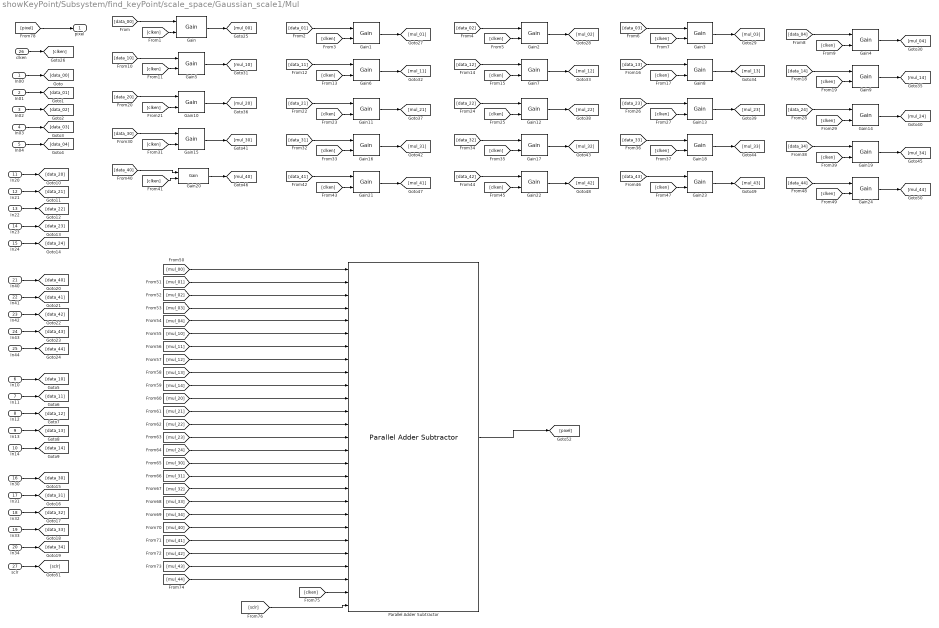
== system showKeyPoint/Subsystem/find_keyPoint/scale_space/Gaussian_scale1/Mul ==
  In00 : Inport
  In01 : Inport  Port=2
  In02 : Inport  Port=3
  In03 : Inport  Port=4
  In04 : Inport  Port=5
  In10 : Inport  Port=6
  In11 : Inport  Port=7
  In12 : Inport  Port=8
  In13 : Inport  Port=9
  In14 : Inport  Port=10
  In20 : Inport  Port=11
  In21 : Inport  Port=12
  In22 : Inport  Port=13
  In23 : Inport  Port=14
  In24 : Inport  Port=15
  In30 : Inport  Port=16
  In31 : Inport  Port=17
  In32 : Inport  Port=18
  In33 : Inport  Port=19
  In34 : Inport  Port=20
  In40 : Inport  Port=21
  In41 : Inport  Port=22
  In42 : Inport  Port=23
  In43 : Inport  Port=24
  In44 : Inport  Port=25
  clken : Inport  Port=26
  sclr : Inport  Port=27
  Gain : allblocks_alteradspbuilder2/Gain  vgain=0.005  BusType=Unsigned Fractional  bwl=8  bwr=16  pipeline=16  pipeline_display=16  allowFloatingPointOverride=on  logOutputs=off  logFile=C:\Users\ASUS\Desktop\sift_fpga_final\Gaussian filter 5x5\tb_gauss\gauss_Subsystem_find%5FkeyPoint_scale%5Fspace_Gaussian%5Fscale1_Mul_Gain.fixedpointlog  use_ena=on  use_aclr=off  lpm=off  MaskValue=1
  Gain1 : allblocks_alteradspbuilder2/Gain  vgain=0.0173  BusType=Unsigned Fractional  bwl=8  bwr=16  pipeline=16  pipeline_display=16  allowFloatingPointOverride=on  logOutputs=off  logFile=C:\Users\ASUS\Desktop\sift_fpga_final\Gaussian filter 5x5\tb_gauss\gauss_Subsystem_find%5FkeyPoint_scale%5Fspace_Gaussian%5Fscale1_Mul_Gain1.fixedpointlog  use_ena=on  use_aclr=off  lpm=off  MaskValue=1
  Gain10 : allblocks_alteradspbuilder2/Gain  vgain=0.0262  BusType=Unsigned Fractional  bwl=8  bwr=16  pipeline=16  pipeline_display=16  allowFloatingPointOverride=on  logOutputs=off  logFile=C:\Users\ASUS\Desktop\sift_fpga_final\Gaussian filter 5x5\tb_gauss\gauss_Subsystem_find%5FkeyPoint_scale%5Fspace_Gaussian%5Fscale1_Mul_Gain10.fixedpointlog  use_ena=on  use_aclr=off  lpm=off  MaskValue=1
  Gain11 : allblocks_alteradspbuilder2/Gain  vgain=0.0903  BusType=Unsigned Fractional  bwl=8  bwr=16  pipeline=16  pipeline_display=16  allowFloatingPointOverride=on  logOutputs=off  logFile=C:\Users\ASUS\Desktop\sift_fpga_final\Gaussian filter 5x5\tb_gauss\gauss_Subsystem_find%5FkeyPoint_scale%5Fspace_Gaussian%5Fscale1_Mul_Gain11.fixedpointlog  use_ena=on  use_aclr=off  lpm=off  MaskValue=1
  Gain12 : allblocks_alteradspbuilder2/Gain  vgain=0.1366  BusType=Unsigned Fractional  bwl=8  bwr=16  pipeline=16  pipeline_display=16  allowFloatingPointOverride=on  logOutputs=off  logFile=C:\Users\ASUS\Desktop\sift_fpga_final\Gaussian filter 5x5\tb_gauss\gauss_Subsystem_find%5FkeyPoint_scale%5Fspace_Gaussian%5Fscale1_Mul_Gain12.fixedpointlog  use_ena=on  use_aclr=off  lpm=off  MaskValue=1
  Gain13 : allblocks_alteradspbuilder2/Gain  vgain=0.0903  BusType=Unsigned Fractional  bwl=8  bwr=16  pipeline=16  pipeline_display=16  allowFloatingPointOverride=on  logOutputs=off  logFile=C:\Users\ASUS\Desktop\sift_fpga_final\Gaussian filter 5x5\tb_gauss\gauss_Subsystem_find%5FkeyPoint_scale%5Fspace_Gaussian%5Fscale1_Mul_Gain13.fixedpointlog  use_ena=on  use_aclr=off  lpm=off  MaskValue=1
  Gain14 : allblocks_alteradspbuilder2/Gain  vgain=0.0262  BusType=Unsigned Fractional  bwl=8  bwr=16  pipeline=16  pipeline_display=16  allowFloatingPointOverride=on  logOutputs=off  logFile=C:\Users\ASUS\Desktop\sift_fpga_final\Gaussian filter 5x5\tb_gauss\gauss_Subsystem_find%5FkeyPoint_scale%5Fspace_Gaussian%5Fscale1_Mul_Gain14.fixedpointlog  use_ena=on  use_aclr=off  lpm=off  MaskValue=1
  Gain15 : allblocks_alteradspbuilder2/Gain  vgain=0.0173  BusType=Unsigned Fractional  bwl=8  bwr=16  pipeline=16  pipeline_display=16  allowFloatingPointOverride=on  logOutputs=off  logFile=C:\Users\ASUS\Desktop\sift_fpga_final\Gaussian filter 5x5\tb_gauss\gauss_Subsystem_find%5FkeyPoint_scale%5Fspace_Gaussian%5Fscale1_Mul_Gain15.fixedpointlog  use_ena=on  use_aclr=off  lpm=off  MaskValue=1
  Gain16 : allblocks_alteradspbuilder2/Gain  vgain=0.0598  BusType=Unsigned Fractional  bwl=8  bwr=16  pipeline=16  pipeline_display=16  allowFloatingPointOverride=on  logOutputs=off  logFile=C:\Users\ASUS\Desktop\sift_fpga_final\Gaussian filter 5x5\tb_gauss\gauss_Subsystem_find%5FkeyPoint_scale%5Fspace_Gaussian%5Fscale1_Mul_Gain16.fixedpointlog  use_ena=on  use_aclr=off  lpm=off  MaskValue=1
  Gain17 : allblocks_alteradspbuilder2/Gain  vgain=0.0903  BusType=Unsigned Fractional  bwl=8  bwr=16  pipeline=16  pipeline_display=16  allowFloatingPointOverride=on  logOutputs=off  logFile=C:\Users\ASUS\Desktop\sift_fpga_final\Gaussian filter 5x5\tb_gauss\gauss_Subsystem_find%5FkeyPoint_scale%5Fspace_Gaussian%5Fscale1_Mul_Gain17.fixedpointlog  use_ena=on  use_aclr=off  lpm=off  MaskValue=1
  Gain18 : allblocks_alteradspbuilder2/Gain  vgain=0.0598  BusType=Unsigned Fractional  bwl=8  bwr=16  pipeline=16  pipeline_display=16  allowFloatingPointOverride=on  logOutputs=off  logFile=C:\Users\ASUS\Desktop\sift_fpga_final\Gaussian filter 5x5\tb_gauss\gauss_Subsystem_find%5FkeyPoint_scale%5Fspace_Gaussian%5Fscale1_Mul_Gain18.fixedpointlog  use_ena=on  use_aclr=off  lpm=off  MaskValue=1
  Gain19 : allblocks_alteradspbuilder2/Gain  vgain=0.0173  BusType=Unsigned Fractional  bwl=8  bwr=16  pipeline=16  pipeline_display=16  allowFloatingPointOverride=on  logOutputs=off  logFile=C:\Users\ASUS\Desktop\sift_fpga_final\Gaussian filter 5x5\tb_gauss\gauss_Subsystem_find%5FkeyPoint_scale%5Fspace_Gaussian%5Fscale1_Mul_Gain19.fixedpointlog  use_ena=on  use_aclr=off  lpm=off  MaskValue=1
  Gain2 : allblocks_alteradspbuilder2/Gain  vgain=0.0262  BusType=Unsigned Fractional  bwl=8  bwr=16  pipeline=16  pipeline_display=16  allowFloatingPointOverride=on  logOutputs=off  logFile=C:\Users\ASUS\Desktop\sift_fpga_final\Gaussian filter 5x5\tb_gauss\gauss_Subsystem_find%5FkeyPoint_scale%5Fspace_Gaussian%5Fscale1_Mul_Gain2.fixedpointlog  use_ena=on  use_aclr=off  lpm=off  MaskValue=1
  Gain20 : allblocks_alteradspbuilder2/Gain  vgain=0.005  BusType=Unsigned Fractional  bwl=8  bwr=16  pipeline=16  pipeline_display=16  allowFloatingPointOverride=on  logOutputs=off  logFile=C:\Users\ASUS\Desktop\sift_fpga_final\Gaussian filter 5x5\tb_gauss\gauss_Subsystem_find%5FkeyPoint_scale%5Fspace_Gaussian%5Fscale1_Mul_Gain20.fixedpointlog  use_ena=on  use_aclr=off  lpm=off  MaskValue=1
  Gain21 : allblocks_alteradspbuilder2/Gain  vgain=0.0173  BusType=Unsigned Fractional  bwl=8  bwr=16  pipeline=16  pipeline_display=16  allowFloatingPointOverride=on  logOutputs=off  logFile=C:\Users\ASUS\Desktop\sift_fpga_final\Gaussian filter 5x5\tb_gauss\gauss_Subsystem_find%5FkeyPoint_scale%5Fspace_Gaussian%5Fscale1_Mul_Gain21.fixedpointlog  use_ena=on  use_aclr=off  lpm=off  MaskValue=1
  Gain22 : allblocks_alteradspbuilder2/Gain  vgain=0.0262  BusType=Unsigned Fractional  bwl=8  bwr=16  pipeline=16  pipeline_display=16  allowFloatingPointOverride=on  logOutputs=off  logFile=C:\Users\ASUS\Desktop\sift_fpga_final\Gaussian filter 5x5\tb_gauss\gauss_Subsystem_find%5FkeyPoint_scale%5Fspace_Gaussian%5Fscale1_Mul_Gain22.fixedpointlog  use_ena=on  use_aclr=off  lpm=off  MaskValue=1
  Gain23 : allblocks_alteradspbuilder2/Gain  vgain=0.0173  BusType=Unsigned Fractional  bwl=8  bwr=16  pipeline=16  pipeline_display=16  allowFloatingPointOverride=on  logOutputs=off  logFile=C:\Users\ASUS\Desktop\sift_fpga_final\Gaussian filter 5x5\tb_gauss\gauss_Subsystem_find%5FkeyPoint_scale%5Fspace_Gaussian%5Fscale1_Mul_Gain23.fixedpointlog  use_ena=on  use_aclr=off  lpm=off  MaskValue=1
  Gain24 : allblocks_alteradspbuilder2/Gain  vgain=0.005  BusType=Unsigned Fractional  bwl=8  bwr=16  pipeline=16  pipeline_display=16  allowFloatingPointOverride=on  logOutputs=off  logFile=C:\Users\ASUS\Desktop\sift_fpga_final\Gaussian filter 5x5\tb_gauss\gauss_Subsystem_find%5FkeyPoint_scale%5Fspace_Gaussian%5Fscale1_Mul_Gain24.fixedpointlog  use_ena=on  use_aclr=off  lpm=off  MaskValue=1
  Gain3 : allblocks_alteradspbuilder2/Gain  vgain=0.0173  BusType=Unsigned Fractional  bwl=8  bwr=16  pipeline=16  pipeline_display=16  allowFloatingPointOverride=on  logOutputs=off  logFile=C:\Users\ASUS\Desktop\sift_fpga_final\Gaussian filter 5x5\tb_gauss\gauss_Subsystem_find%5FkeyPoint_scale%5Fspace_Gaussian%5Fscale1_Mul_Gain3.fixedpointlog  use_ena=on  use_aclr=off  lpm=off  MaskValue=1
  Gain4 : allblocks_alteradspbuilder2/Gain  vgain=0.005  BusType=Unsigned Fractional  bwl=8  bwr=16  pipeline=16  pipeline_display=16  allowFloatingPointOverride=on  logOutputs=off  logFile=C:\Users\ASUS\Desktop\sift_fpga_final\Gaussian filter 5x5\tb_gauss\gauss_Subsystem_find%5FkeyPoint_scale%5Fspace_Gaussian%5Fscale1_Mul_Gain4.fixedpointlog  use_ena=on  use_aclr=off  lpm=off  MaskValue=1
  Gain5 : allblocks_alteradspbuilder2/Gain  vgain=0.0173  BusType=Unsigned Fractional  bwl=8  bwr=16  pipeline=16  pipeline_display=16  allowFloatingPointOverride=on  logOutputs=off  logFile=C:\Users\ASUS\Desktop\sift_fpga_final\Gaussian filter 5x5\tb_gauss\gauss_Subsystem_find%5FkeyPoint_scale%5Fspace_Gaussian%5Fscale1_Mul_Gain5.fixedpointlog  use_ena=on  use_aclr=off  lpm=off  MaskValue=1
  Gain6 : allblocks_alteradspbuilder2/Gain  vgain=0.0598  BusType=Unsigned Fractional  bwl=8  bwr=16  pipeline=16  pipeline_display=16  allowFloatingPointOverride=on  logOutputs=off  logFile=C:\Users\ASUS\Desktop\sift_fpga_final\Gaussian filter 5x5\tb_gauss\gauss_Subsystem_find%5FkeyPoint_scale%5Fspace_Gaussian%5Fscale1_Mul_Gain6.fixedpointlog  use_ena=on  use_aclr=off  lpm=off  MaskValue=1
  Gain7 : allblocks_alteradspbuilder2/Gain  vgain=0.0903  BusType=Unsigned Fractional  bwl=8  bwr=16  pipeline=16  pipeline_display=16  allowFloatingPointOverride=on  logOutputs=off  logFile=C:\Users\ASUS\Desktop\sift_fpga_final\Gaussian filter 5x5\tb_gauss\gauss_Subsystem_find%5FkeyPoint_scale%5Fspace_Gaussian%5Fscale1_Mul_Gain7.fixedpointlog  use_ena=on  use_aclr=off  lpm=off  MaskValue=1
  Gain8 : allblocks_alteradspbuilder2/Gain  vgain=0.0598  BusType=Unsigned Fractional  bwl=8  bwr=16  pipeline=16  pipeline_display=16  allowFloatingPointOverride=on  logOutputs=off  logFile=C:\Users\ASUS\Desktop\sift_fpga_final\Gaussian filter 5x5\tb_gauss\gauss_Subsystem_find%5FkeyPoint_scale%5Fspace_Gaussian%5Fscale1_Mul_Gain8.fixedpointlog  use_ena=on  use_aclr=off  lpm=off  MaskValue=1
  Gain9 : allblocks_alteradspbuilder2/Gain  vgain=0.0173  BusType=Unsigned Fractional  bwl=8  bwr=16  pipeline=16  pipeline_display=16  allowFloatingPointOverride=on  logOutputs=off  logFile=C:\Users\ASUS\Desktop\sift_fpga_final\Gaussian filter 5x5\tb_gauss\gauss_Subsystem_find%5FkeyPoint_scale%5Fspace_Gaussian%5Fscale1_Mul_Gain9.fixedpointlog  use_ena=on  use_aclr=off  lpm=off  MaskValue=1
  Parallel Adder Subtractor : allblocks_alteradspbuilder2/Parallel Adder Subtractor  number_of_inputs=25  direction=+  use_pipeline=on  pipeline_display=5  phase_selection=1  use_ena=on  use_aclr=on  allowFloatingPointOverride=on  logOutputs=off  logFile=C:\Users\ASUS\Desktop\sift_fpga_final\Gaussian filter 5x5\tb_gauss\gauss_Subsystem_find%5FkeyPoint_scale%5Fspace_Gaussian%5Fscale1_Mul_Parallel+Adder+Subtractor.fixedpointlog
  pixel : Outport
  wires:
  In00/1 -> [data_00]
  In21/1 -> [data_21]
  In30/1 -> [data_30]
  In04/1 -> [data_04]
  In03/1 -> [data_03]
  In14/1 -> [data_14]
  In02/1 -> [data_02]
  In13/1 -> [data_13]
  In31/1 -> [data_31]
  In20/1 -> [data_20]
  In22/1 -> [data_22]
  In24/1 -> [data_24]
  In23/1 -> [data_23]
  In01/1 -> [data_01]
  In32/1 -> [data_32]
  In34/1 -> [data_34]
  In33/1 -> [data_33]
  In40/1 -> [data_40]
  In41/1 -> [data_41]
  In42/1 -> [data_42]
  In44/1 -> [data_44]
  In12/1 -> [data_12]
  In11/1 -> [data_11]
  In10/1 -> [data_10]
  Gain1/1 -> [mul_01]
  Gain4/1 -> [mul_04]
  [clken] -> Gain1/2
  [data_11] -> Gain6/1
  Gain6/1 -> [mul_11]
  [data_12] -> Gain7/1
  [clken] -> Gain4/2
  Gain2/1 -> [mul_02]
  [data_01] -> Gain1/1
  [data_04] -> Gain4/1
  [clken] -> Gain6/2
  Gain3/1 -> [mul_03]
  clken/1 -> [clken]
  [clken] -> Gain7/2
  [data_02] -> Gain2/1
  [data_03] -> Gain3/1
  [data_00] -> Gain/1
  Gain5/1 -> [mul_10]
  Gain/1 -> [mul_00]
  [clken] -> Gain3/2
  [data_10] -> Gain5/1
  In43/1 -> [data_43]
  [clken] -> Gain2/2
  [clken] -> Gain5/2
  [clken] -> Gain13/2
  [clken] -> Gain15/2
  [data_22] -> Gain12/1
  [clken] -> Gain8/2
  [data_20] -> Gain10/1
  [clken] -> Gain9/2
  Gain9/1 -> [mul_14]
  Gain10/1 -> [mul_20]
  [clken] -> Gain11/2
  Gain11/1 -> [mul_21]
  [clken] -> Gain10/2
  [data_14] -> Gain9/1
  Gain13/1 -> [mul_23]
  [clken] -> Gain14/2
  Gain7/1 -> [mul_12]
  [data_13] -> Gain8/1
  [clken] -> Gain12/2
  Gain8/1 -> [mul_13]
  Gain12/1 -> [mul_22]
  [data_24] -> Gain14/1
  [data_23] -> Gain13/1
  Gain14/1 -> [mul_24]
  [data_30] -> Gain15/1
  [data_21] -> Gain11/1
  Gain16/1 -> [mul_31]
  [data_34] -> Gain19/1
  [clken] -> Gain20/2
  [clken] -> Gain19/2
  Gain17/1 -> [mul_32]
  Gain18/1 -> [mul_33]
  Gain20/1 -> [mul_40]
  [clken] -> Gain17/2
  [clken] -> Gain21/2
  [data_31] -> Gain16/1
  [data_33] -> Gain18/1
  [clken] -> Gain16/2
  Gain19/1 -> [mul_34]
  [data_42] -> Gain22/1
  Gain21/1 -> [mul_41]
  Gain22/1 -> [mul_42]
  [data_43] -> Gain23/1
  [clken] -> Gain23/2
  Gain15/1 -> [mul_30]
  [clken] -> Gain18/2
  [data_40] -> Gain20/1
  [data_32] -> Gain17/1
  [data_41] -> Gain21/1
  [clken] -> Gain22/2
  Gain24/1 -> [mul_44]
  [clken] -> Gain24/2
  [data_44] -> Gain24/1
  Gain23/1 -> [mul_43]
  [clken] -> Gain/2
  Parallel Adder Subtractor/1 -> [pixel]
  [pixel] -> pixel/1
  [mul_00] -> Parallel Adder Subtractor/1
  [mul_01] -> Parallel Adder Subtractor/2
  [mul_02] -> Parallel Adder Subtractor/3
  [mul_03] -> Parallel Adder Subtractor/4
  [mul_04] -> Parallel Adder Subtractor/5
  [mul_10] -> Parallel Adder Subtractor/6
  [mul_11] -> Parallel Adder Subtractor/7
  [mul_12] -> Parallel Adder Subtractor/8
  [mul_13] -> Parallel Adder Subtractor/9
  [mul_14] -> Parallel Adder Subtractor/10
  [mul_20] -> Parallel Adder Subtractor/11
  [mul_21] -> Parallel Adder Subtractor/12
  [mul_22] -> Parallel Adder Subtractor/13
  [mul_23] -> Parallel Adder Subtractor/14
  [mul_24] -> Parallel Adder Subtractor/15
  [mul_31] -> Parallel Adder Subtractor/17
  [mul_32] -> Parallel Adder Subtractor/18
  [mul_33] -> Parallel Adder Subtractor/19
  [mul_34] -> Parallel Adder Subtractor/20
  [mul_40] -> Parallel Adder Subtractor/21
  [mul_41] -> Parallel Adder Subtractor/22
  [mul_42] -> Parallel Adder Subtractor/23
  [mul_43] -> Parallel Adder Subtractor/24
  [mul_44] -> Parallel Adder Subtractor/25
  [mul_30] -> Parallel Adder Subtractor/16
  [clken] -> Parallel Adder Subtractor/26
  sclr/1 -> [sclr]
  [sclr] -> Parallel Adder Subtractor/27
